simulink model "L2_T5_position_loop"  (R2026a)
settings: Solver=ode23tb  StartTime=0  StopTime=0.3  MaxStep=5e-05
settings Model: Creator=m  LastModifiedBy=m

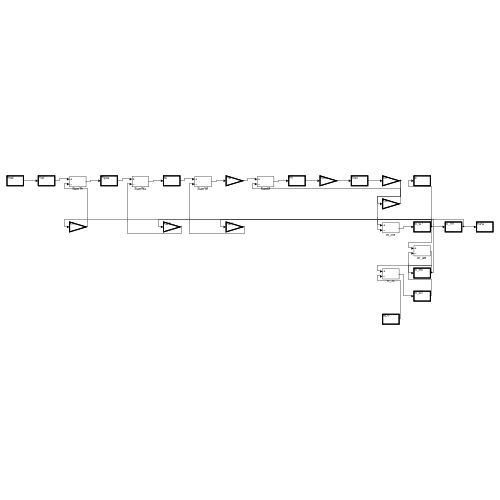
[thumbnail: Simulink's stored preview of the top-level diagram]
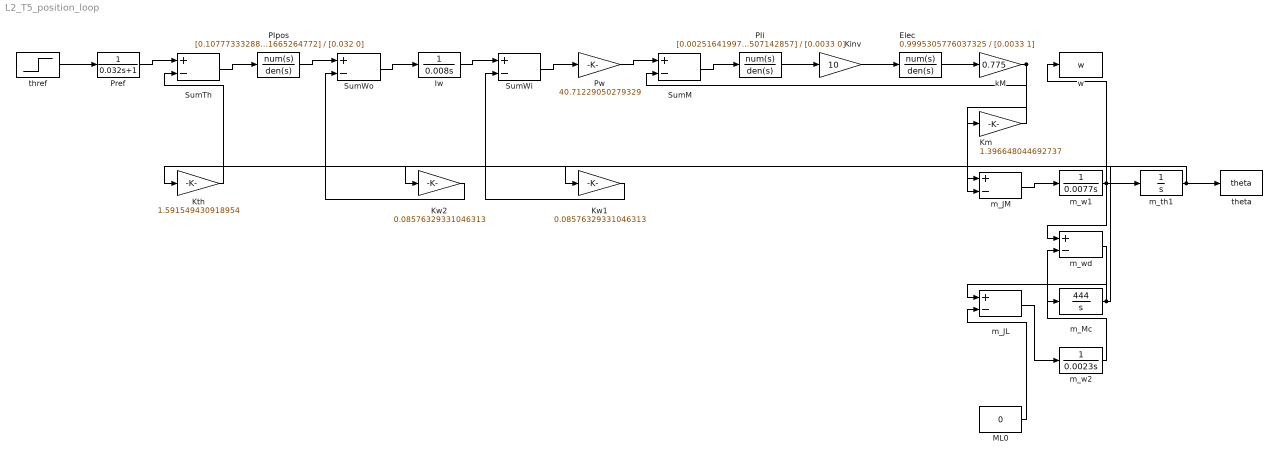
== system L2_T5_position_loop ==
  Elec : TransferFcn  Numerator=0.9995305776037325  Denominator=[0.0033 1]
  Iw : TransferFcn  Numerator=1  Denominator=[0.008 0]
  Kinv : Gain  Gain=10
  Km : Gain  Gain=1.396648044692737
  Kth : Gain  Gain=1.591549430918954
  Kw1 : Gain  Gain=0.08576329331046313
  Kw2 : Gain  Gain=0.08576329331046313
  ML0 : Constant  Value=0
  PIi : TransferFcn  Numerator=[0.002516419973571428 0.762551507142857]  Denominator=[0.0033 0]
  PIpos : TransferFcn  Numerator=[0.107773332884727 3.36791665264772]  Denominator=[0.032 0]
  Pref : TransferFcn  Numerator=1  Denominator=[0.032 1]
  Pw : Gain  Gain=40.71229050279329
  SumM : Sum  Inputs=+-
  SumTh : Sum  Inputs=+-
  SumWi : Sum  Inputs=+-
  SumWo : Sum  Inputs=+-
  kM : Gain  Gain=0.775
  m_JL : Sum  Inputs=+-
  m_JM : Sum  Inputs=+-
  m_Mc : TransferFcn  Numerator=444  Denominator=[1 0]
  m_th1 : Integrator
  m_w1 : TransferFcn  Numerator=1  Denominator=[0.0077 0]
  m_w2 : TransferFcn  Numerator=1  Denominator=[0.0023 0]
  m_wd : Sum  Inputs=+-
  theta : ToWorkspace  VariableName=theta  SaveFormat=Structure With Time  SampleTime=-1
  thref : Step  Time=0  FinalValue=2.5  SampleTime=0
  w : ToWorkspace  VariableName=w  SaveFormat=Structure With Time  SampleTime=-1
  wires:
  m_JM/1 -> m_w1/1
  m_w1/1 -> m_wd/1, m_th1/1, Kw1/1, Kw2/1, w/1
  m_w2/1 -> m_wd/2
  m_wd/1 -> m_Mc/1
  m_Mc/1 -> m_JM/2, m_JL/1
  m_JL/1 -> m_w2/1
  thref/1 -> Pref/1
  Pref/1 -> SumTh/1
  SumTh/1 -> PIpos/1
  PIpos/1 -> SumWo/1
  SumWo/1 -> Iw/1
  Iw/1 -> SumWi/1
  SumWi/1 -> Pw/1
  Pw/1 -> SumM/1
  SumM/1 -> PIi/1
  PIi/1 -> Kinv/1
  Kinv/1 -> Elec/1
  Elec/1 -> kM/1
  kM/1 -> m_JM/1, Km/1
  ML0/1 -> m_JL/2
  Km/1 -> SumM/2
  Kw1/1 -> SumWi/2
  Kw2/1 -> SumWo/2
  m_th1/1 -> Kth/1, theta/1
  Kth/1 -> SumTh/2
